simulink model "first_3phase_multilevel_doros"  (R2015a)
settings: Solver=ode45  StartTime=0.02  StopTime=0.04  RelTol=1e-3
libraries: simulink x85, powerlib_meascontrol x77, powerlib x52
settings Model: Creator=yahya  LastModifiedBy=Yahya

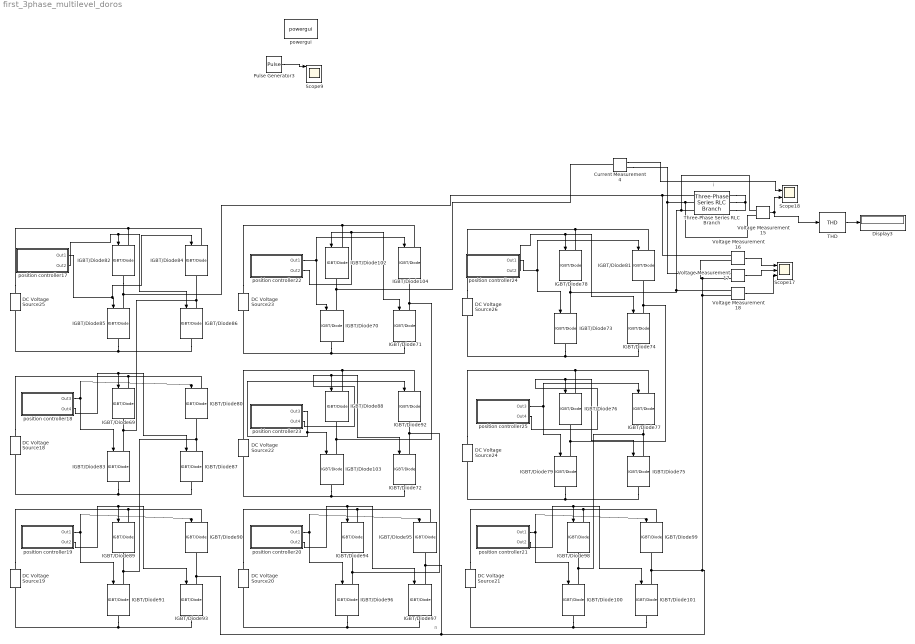
== system first_3phase_multilevel_doros ==
  note: n
  note: i
  Current Measurement4 : powerlib/Measurements/Current Measurement  PhasorSimulation=off  OutputType=Complex  PSBequivalent=0
  DC Voltage Source{18..26} (9 alike) : powerlib/Electrical Sources/DC Voltage Source  Amplitude=100  Measurements=None
  Display3 : Display
  IGBT/Diode{69..104} (36 alike) : powerlib/Power Electronics/IGBT//Diode  Ron=1e-3  Rs=1e5  Cs=inf  Measurements=off
  Pulse Generator3 : DiscretePulseGenerator  PulseType=Time based  Amplitude=0.8  Period=0.00001  PulseWidth=50
  Scope17 : Scope  NumInputPorts=3
      settings: TimeRange=0.02  YMin=-5~-5~-5  YMax=5~5~5  SaveName=ScopeData15
  Scope18 : Scope  NumInputPorts=2
      settings: TimeRange=1  YMin=-400~-400  YMax=400~400  SaveName=ScopeData16
  Scope9 : Scope  NumInputPorts=4
      settings: YMin=-5~-5~-5~-5  YMax=5~5~5~5  SaveName=ScopeData18
  THD : powerlib_meascontrol/Measurements/THD  Freq=50  Ts=0
  Three-Phase Series RLC Branch : powerlib/Elements/Three-Phase Series RLC Branch  LConnTagsString=A|B|C  RConnTagsString=A|B|C  BranchType=RL  Resistance=2.81  Inductance=0.01167  Capacitance=1e-6  Measurements=None
  Voltage Measurement{15..18} (4 alike) : powerlib/Measurements/Voltage Measurement  PhasorSimulation=off  OutputType=Complex  PSBequivalent=0
  position controller17 : Subsystem
  position controller18 : Subsystem
  position controller19 : Subsystem
  position controller20 : Subsystem
  position controller21 : Subsystem
  position controller22 : Subsystem
  position controller23 : Subsystem
  position controller24 : Subsystem
  position controller25 : Subsystem
  powergui : powerlib/powergui  Priority=1  SimulationMode=Continuous  SolverType=Tustin/Backward Euler (TBE)  SampleTime=50e-6  frequency=60  SPID=off  DisableSnubberDevices=off  DisableRonSwitches=off  DisableVfSwitches=off  SwTol=0  DisplayEquations=off  Interpol=off  methode=off  Ts=100  FunctionMessages=off  echomessages=off  HookPort=off  EnableUseOfTLC=off  x0status=blocks  frequencyindice=0  Pbase=100e6  ErrMax=1e-4  Iterations=50  UnitsV=kV  UnitsW=MW  buscounter=0  RestoreLinks=warning  ResistiveCurrentMeasurement=off  Frange=[0:2:500]  Ylog=off  Xlog=on  ShowGrid=off  save=off  variable=ZData  structure=0  ZoomFFT=off  StartTime=0.0  cycles=1  DisplayStyle=1  fundamental=60  FreqAxis=off  MaxFrequency=1000  frequencyindicesteady=1  RmsSteady=1  display=off
  wires:
  position controller17/2(Out2) -> IGBT/Diode86/1, IGBT/Diode82/1
  Pulse Generator3/1 -> Scope9/1
  Current Measurement4/1 -> Scope18/1
  position controller17/1(Out1) -> IGBT/Diode85/1, IGBT/Diode84/1
  position controller18/2(Out4) -> IGBT/Diode87/1, IGBT/Diode69/1
  position controller18/1(Out3) -> IGBT/Diode83/1, IGBT/Diode80/1
  position controller22/2(Out2) -> IGBT/Diode102/1, IGBT/Diode71/1
  position controller22/1(Out1) -> IGBT/Diode70/1, IGBT/Diode104/1
  position controller23/2(Out4) -> IGBT/Diode72/1, IGBT/Diode88/1
  position controller23/1(Out3) -> IGBT/Diode103/1, IGBT/Diode92/1
  position controller24/2(Out2) -> IGBT/Diode74/1, IGBT/Diode78/1
  position controller24/1(Out1) -> IGBT/Diode81/1, IGBT/Diode73/1
  position controller25/2(Out4) -> IGBT/Diode75/1, IGBT/Diode76/1
  position controller25/1(Out3) -> IGBT/Diode79/1, IGBT/Diode77/1
  Voltage Measurement15/1 -> Scope18/2, THD/1
  Voltage Measurement16/1 -> Scope17/1
  Voltage Measurement17/1 -> Scope17/2
  Voltage Measurement18/1 -> Scope17/3
  position controller19/2(Out2) -> IGBT/Diode93/1, IGBT/Diode89/1
  position controller19/1(Out1) -> IGBT/Diode91/1, IGBT/Diode90/1
  position controller20/2(Out2) -> IGBT/Diode97/1, IGBT/Diode94/1
  position controller20/1(Out1) -> IGBT/Diode96/1, IGBT/Diode95/1
  position controller21/2(Out2) -> IGBT/Diode101/1, IGBT/Diode98/1
  position controller21/1(Out1) -> IGBT/Diode100/1, IGBT/Diode99/1
  THD/1 -> Display3/1
  connections:
  DC Voltage Source25/RConn1 -- IGBT/Diode84/LConn1 -- IGBT/Diode82/LConn1
  DC Voltage Source25/LConn1 -- IGBT/Diode85/RConn1 -- IGBT/Diode86/RConn1
  IGBT/Diode84/RConn1 -- IGBT/Diode86/LConn1 -- IGBT/Diode69/RConn1 -- IGBT/Diode83/LConn1
  DC Voltage Source18/RConn1 -- IGBT/Diode80/LConn1 -- IGBT/Diode69/LConn1
  DC Voltage Source18/LConn1 -- IGBT/Diode87/RConn1 -- IGBT/Diode83/RConn1
  DC Voltage Source23/RConn1 -- IGBT/Diode104/LConn1 -- IGBT/Diode102/LConn1
  DC Voltage Source23/LConn1 -- IGBT/Diode71/RConn1 -- IGBT/Diode70/RConn1
  IGBT/Diode102/RConn1 -- Current Measurement4/LConn1 -- IGBT/Diode70/LConn1
  IGBT/Diode92/LConn1 -- DC Voltage Source22/RConn1 -- IGBT/Diode88/LConn1
  DC Voltage Source22/LConn1 -- IGBT/Diode72/RConn1 -- IGBT/Diode103/RConn1
  IGBT/Diode88/RConn1 -- IGBT/Diode103/LConn1 -- IGBT/Diode71/LConn1 -- IGBT/Diode104/RConn1
  DC Voltage Source26/RConn1 -- IGBT/Diode81/LConn1 -- IGBT/Diode78/LConn1
  DC Voltage Source26/LConn1 -- IGBT/Diode74/RConn1 -- IGBT/Diode73/RConn1
  DC Voltage Source24/RConn1 -- IGBT/Diode77/LConn1 -- IGBT/Diode76/LConn1
  DC Voltage Source24/LConn1 -- IGBT/Diode75/RConn1 -- IGBT/Diode79/RConn1
  IGBT/Diode74/LConn1 -- IGBT/Diode81/RConn1 -- IGBT/Diode76/RConn1 -- IGBT/Diode79/LConn1
  IGBT/Diode73/LConn1 -- Voltage Measurement15/LConn1 -- Three-Phase Series RLC Branch/LConn3 -- Voltage Measurement18/LConn1 -- IGBT/Diode78/RConn1
  IGBT/Diode82/RConn1 -- Three-Phase Series RLC Branch/LConn1 -- Voltage Measurement16/LConn1 -- IGBT/Diode85/LConn1
  Three-Phase Series RLC Branch/RConn2 -- Three-Phase Series RLC Branch/RConn3 -- Three-Phase Series RLC Branch/RConn1
  IGBT/Diode89/RConn1 -- IGBT/Diode91/LConn1 -- IGBT/Diode80/RConn1 -- IGBT/Diode87/LConn1
  IGBT/Diode94/RConn1 -- IGBT/Diode96/LConn1 -- IGBT/Diode92/RConn1 -- IGBT/Diode72/LConn1
  IGBT/Diode98/RConn1 -- IGBT/Diode100/LConn1 -- IGBT/Diode77/RConn1 -- IGBT/Diode75/LConn1
  DC Voltage Source19/RConn1 -- IGBT/Diode90/LConn1 -- IGBT/Diode89/LConn1
  DC Voltage Source19/LConn1 -- IGBT/Diode93/RConn1 -- IGBT/Diode91/RConn1
  DC Voltage Source20/RConn1 -- IGBT/Diode95/LConn1 -- IGBT/Diode94/LConn1
  DC Voltage Source20/LConn1 -- IGBT/Diode97/RConn1 -- IGBT/Diode96/RConn1
  DC Voltage Source21/RConn1 -- IGBT/Diode99/LConn1 -- IGBT/Diode98/LConn1
  DC Voltage Source21/LConn1 -- IGBT/Diode101/RConn1 -- IGBT/Diode100/RConn1
  IGBT/Diode93/LConn1 -- IGBT/Diode90/RConn1 -- Voltage Measurement16/LConn2 -- Voltage Measurement17/LConn2 -- Voltage Measurement18/LConn2 -- IGBT/Diode99/RConn1 -- IGBT/Diode101/LConn1 -- IGBT/Diode95/RConn1 -- IGBT/Diode97/LConn1
  Three-Phase Series RLC Branch/LConn2 -- Voltage Measurement17/LConn1 -- Current Measurement4/RConn1 -- Voltage Measurement15/LConn2

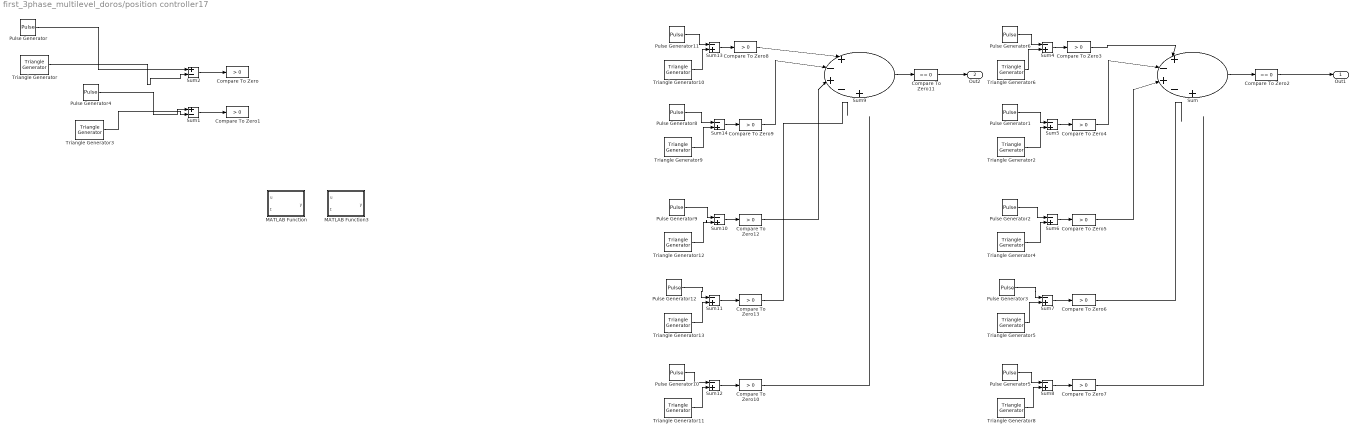
== system first_3phase_multilevel_doros/position controller17 ==
  Compare To Zero{,1,3..10,12..13} (12 alike) : simulink/Logic and Bit Operations/Compare To Zero  relop=>  OutDataTypeStr=boolean  ZeroCross=off
  Compare To Zero11 : simulink/Logic and Bit Operations/Compare To Zero  relop===  OutDataTypeStr=boolean  ZeroCross=off
  Compare To Zero2 : simulink/Logic and Bit Operations/Compare To Zero  relop===  OutDataTypeStr=boolean  ZeroCross=off
  MATLAB Function : MATLAB Function  TreatAsAtomicUnit=on
  MATLAB Function3 : MATLAB Function  TreatAsAtomicUnit=on
  Pulse Generator : DiscretePulseGenerator  PulseType=Time based  Amplitude=0.648099859976388  Period=0.02  PulseWidth=50.001
  Pulse Generator1 : DiscretePulseGenerator  PulseType=Time based  Amplitude=0.687674739965695  Period=0.02  PulseWidth=50.001
  Pulse Generator10 : DiscretePulseGenerator  PulseType=Time based  Amplitude=0.377812988041322  Period=0.02  PulseWidth=50.001  PhaseDelay=0.01
  Pulse Generator11 : DiscretePulseGenerator  PulseType=Time based  Amplitude=0.5150  Period=0.02  PulseWidth=50.001  PhaseDelay=0.01
  Pulse Generator12 : DiscretePulseGenerator  PulseType=Time based  Amplitude=0.360085258924687  Period=0.02  PulseWidth=50.001  PhaseDelay=0.01
  Pulse Generator2 : DiscretePulseGenerator  PulseType=Time based  Amplitude=0.796099800558993  Period=0.02  PulseWidth=50.001
  Pulse Generator3 : DiscretePulseGenerator  PulseType=Time based  Amplitude=0.360085258924687  Period=0.02  PulseWidth=50.001
  Pulse Generator4 : DiscretePulseGenerator  PulseType=Time based  Amplitude=0.648099859976388  Period=0.02  PulseWidth=50.001  PhaseDelay=0.01
  Pulse Generator5 : DiscretePulseGenerator  PulseType=Time based  Amplitude=0.377812988041322  Period=0.02  PulseWidth=50.001
  Pulse Generator6 : DiscretePulseGenerator  PulseType=Time based  Amplitude=0.5150  Period=0.02  PulseWidth=50.001
  Pulse Generator8 : DiscretePulseGenerator  PulseType=Time based  Amplitude=0.687674739965695  Period=0.02  PulseWidth=50.001  PhaseDelay=0.01
  Pulse Generator9 : DiscretePulseGenerator  PulseType=Time based  Amplitude=0.796099800558993  Period=0.02  PulseWidth=50.001  PhaseDelay=0.01
  Sum : Sum  Inputs=|+-+-+
  Sum1 : Sum  Inputs=+-  OutDataTypeStr=double
  Sum{4..8,10..14} (10 alike) : Sum  Inputs=-+  OutDataTypeStr=double
  Sum2 : Sum  Inputs=+-  OutDataTypeStr=double
  Sum9 : Sum  Inputs=|+-+-+
  Triangle Generator{,2,4..6,8} (6 alike) : powerlib_meascontrol/Pulse & Signal Generators/Triangle Generator  Freq=50  Phase=90  Ts=0
  Triangle Generator{3,9..13} (6 alike) : powerlib_meascontrol/Pulse & Signal Generators/Triangle Generator  Freq=50  Phase=90+180  Ts=0
  Out1 : Outport
  Out2 : Outport  Port=2
  wires:
  Pulse Generator/1 -> Sum2/1
  Triangle Generator/1 -> Sum2/2
  Pulse Generator4/1 -> Sum1/1
  Triangle Generator3/1 -> Sum1/2
  Sum2/1 -> Compare To Zero/1
  Sum1/1 -> Compare To Zero1/1
  Triangle Generator6/1 -> Sum4/2
  Sum4/1 -> Compare To Zero3/1
  Pulse Generator6/1 -> Sum4/1
  Triangle Generator2/1 -> Sum5/2
  Sum5/1 -> Compare To Zero4/1
  Pulse Generator1/1 -> Sum5/1
  Triangle Generator4/1 -> Sum6/2
  Sum6/1 -> Compare To Zero5/1
  Pulse Generator2/1 -> Sum6/1
  Triangle Generator5/1 -> Sum7/2
  Sum7/1 -> Compare To Zero6/1
  Pulse Generator3/1 -> Sum7/1
  Triangle Generator8/1 -> Sum8/2
  Sum8/1 -> Compare To Zero7/1
  Pulse Generator5/1 -> Sum8/1
  Compare To Zero3/1 -> Sum/1
  Compare To Zero5/1 -> Sum/3
  Compare To Zero6/1 -> ?
  Compare To Zero7/1 -> ?
  Triangle Generator10/1 -> Sum13/2
  Sum13/1 -> Compare To Zero8/1
  Pulse Generator11/1 -> Sum13/1
  Triangle Generator9/1 -> Sum14/2
  Sum14/1 -> Compare To Zero9/1
  Pulse Generator8/1 -> Sum14/1
  Triangle Generator12/1 -> Sum10/2
  Sum10/1 -> Compare To Zero12/1
  Pulse Generator9/1 -> Sum10/1
  Triangle Generator13/1 -> Sum11/2
  Sum11/1 -> Compare To Zero13/1
  Pulse Generator12/1 -> Sum11/1
  Triangle Generator11/1 -> Sum12/2
  Sum12/1 -> Compare To Zero10/1
  Pulse Generator10/1 -> Sum12/1
  Compare To Zero8/1 -> Sum9/1
  Compare To Zero9/1 -> Sum9/2
  Compare To Zero12/1 -> Sum9/3
  Sum9/1 -> Compare To Zero11/1
  Compare To Zero13/1 -> ?
  Compare To Zero10/1 -> ?
  Compare To Zero4/1 -> Sum/2
  Sum/1 -> Compare To Zero2/1
  Compare To Zero2/1 -> Out1/1
  Compare To Zero11/1 -> Out2/1

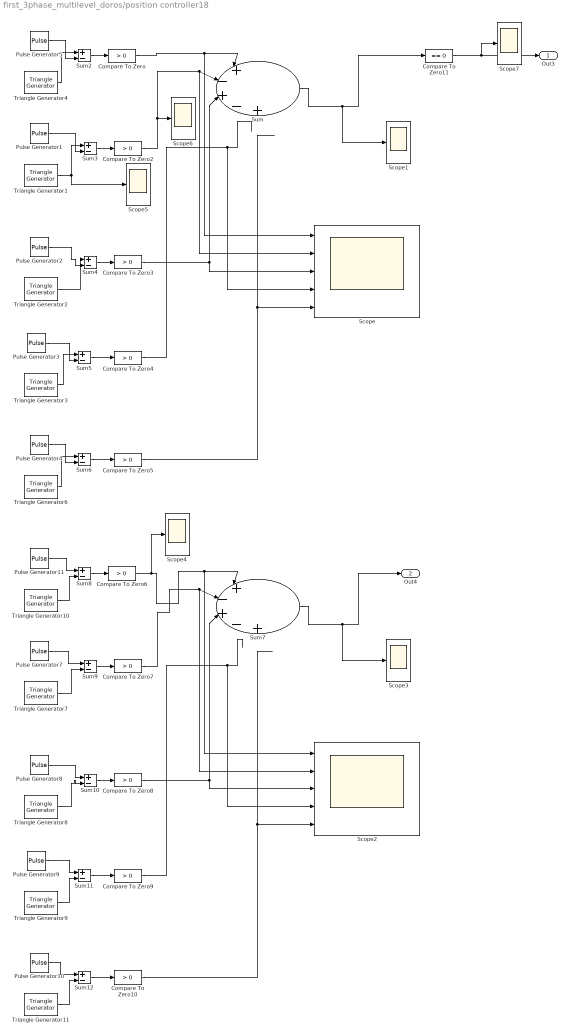
== system first_3phase_multilevel_doros/position controller18 ==
  Compare To Zero{,2..10} (10 alike) : simulink/Logic and Bit Operations/Compare To Zero  relop=>  OutDataTypeStr=boolean  ZeroCross=off
  Compare To Zero11 : simulink/Logic and Bit Operations/Compare To Zero  relop===  OutDataTypeStr=boolean  ZeroCross=off
  Pulse Generator1 : DiscretePulseGenerator  PulseType=Time based  Amplitude=0.372911525752630  Period=0.02  PulseWidth=50.001
  Pulse Generator10 : DiscretePulseGenerator  PulseType=Time based  Amplitude=0.377812988041322  Period=0.02  PulseWidth=50.001  PhaseDelay=0.01
  Pulse Generator11 : DiscretePulseGenerator  PulseType=Time based  Amplitude=0.3014  Period=0.02  PulseWidth=50.001  PhaseDelay=0.01
  Pulse Generator2 : DiscretePulseGenerator  PulseType=Time based  Amplitude=0.399283235379700  Period=0.02  PulseWidth=50.001
  Pulse Generator3 : DiscretePulseGenerator  PulseType=Time based  Amplitude=0.360085258924687  Period=0.02  PulseWidth=50.001
  Pulse Generator4 : DiscretePulseGenerator  PulseType=Time based  Amplitude=0.377812988041322  Period=0.02  PulseWidth=50.001
  Pulse Generator5 : DiscretePulseGenerator  PulseType=Time based  Amplitude=0.3014  Period=0.02  PulseWidth=50.001
  Pulse Generator7 : DiscretePulseGenerator  PulseType=Time based  Amplitude=0.372911525752630  Period=0.02  PulseWidth=50.001  PhaseDelay=0.01
  Pulse Generator8 : DiscretePulseGenerator  PulseType=Time based  Amplitude=0.399283235379700  Period=0.02  PulseWidth=50.001  PhaseDelay=0.01
  Pulse Generator9 : DiscretePulseGenerator  PulseType=Time based  Amplitude=0.360085258924687  Period=0.02  PulseWidth=50.001  PhaseDelay=0.01
  Scope : Scope  NumInputPorts=5
      settings: TimeRange=0.02  YMin=0~0~0~0~0  YMax=1~1~1~1~1  SaveName=ScopeData8
  Scope{1,3..7} (6 alike) : Scope
      Scope1 settings: SaveName=ScopeData17
      Scope3 settings: SaveName=ScopeData45
      Scope4 settings: SaveName=ScopeData46
      Scope5 settings: SaveName=ScopeData47
      Scope6 settings: SaveName=ScopeData48
      Scope7 settings: SaveName=ScopeData49
  Scope2 : Scope  NumInputPorts=5
      settings: YMin=-5~-5~-5~-5~-5  YMax=5~5~5~5~5  SaveName=ScopeData44
  Sum : Sum  Inputs=|+-+-+
  Sum{2..6,8..12} (10 alike) : Sum  Inputs=+-  OutDataTypeStr=double
  Sum7 : Sum  Inputs=|+-+-+
  Triangle Generator{1..4,6} (5 alike) : powerlib_meascontrol/Pulse & Signal Generators/Triangle Generator  Freq=50  Phase=90  Ts=0
  Triangle Generator{7..11} (5 alike) : powerlib_meascontrol/Pulse & Signal Generators/Triangle Generator  Freq=50  Phase=90+180  Ts=0
  Out3 : Outport
  Out4 : Outport  Port=2
  wires:
  Triangle Generator4/1 -> Sum2/1
  Sum2/1 -> Compare To Zero/1
  Pulse Generator5/1 -> Sum2/2
  Triangle Generator1/1 -> Sum3/1, Scope5/1
  Sum3/1 -> Compare To Zero2/1
  Pulse Generator1/1 -> Sum3/2
  Triangle Generator2/1 -> Sum4/1
  Sum4/1 -> Compare To Zero3/1
  Pulse Generator2/1 -> Sum4/2
  Triangle Generator3/1 -> Sum5/1
  Sum5/1 -> Compare To Zero4/1
  Pulse Generator3/1 -> Sum5/2
  Triangle Generator6/1 -> Sum6/1
  Sum6/1 -> Compare To Zero5/1
  Pulse Generator4/1 -> Sum6/2
  Compare To Zero/1 -> Scope/1, Sum/1
  Compare To Zero3/1 -> Sum/3, Scope/3
  Sum/1 -> Scope1/1, Compare To Zero11/1
  Compare To Zero4/1 -> Scope/4
  Compare To Zero5/1 -> Scope/5
  Triangle Generator10/1 -> Sum8/2
  Sum8/1 -> Compare To Zero6/1
  Pulse Generator11/1 -> Sum8/1
  Triangle Generator7/1 -> Sum9/2
  Sum9/1 -> Compare To Zero7/1
  Pulse Generator7/1 -> Sum9/1
  Triangle Generator8/1 -> Sum10/2
  Sum10/1 -> Compare To Zero8/1
  Pulse Generator8/1 -> Sum10/1
  Triangle Generator9/1 -> Sum11/2
  Sum11/1 -> Compare To Zero9/1
  Pulse Generator9/1 -> Sum11/1
  Triangle Generator11/1 -> Sum12/2
  Sum12/1 -> Compare To Zero10/1
  Pulse Generator10/1 -> Sum12/1
  Compare To Zero6/1 -> Scope4/1, Scope2/1, Sum7/1
  Compare To Zero7/1 -> Sum7/2, Scope2/2
  Compare To Zero8/1 -> Sum7/3, Scope2/3
  Sum7/1 -> Out4/1, Scope3/1
  Compare To Zero9/1 -> Scope2/4
  Compare To Zero10/1 -> Scope2/5
  Compare To Zero2/1 -> Sum/2, Scope/2, Scope6/1
  Compare To Zero11/1 -> Scope7/1, Out3/1

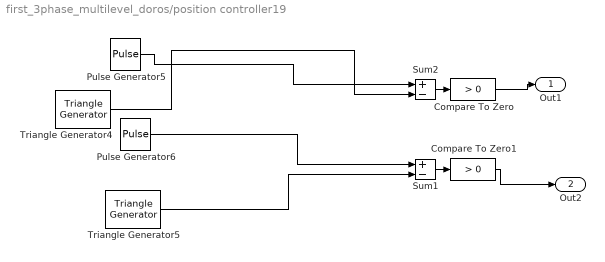
== system first_3phase_multilevel_doros/position controller19 ==
  Compare To Zero : simulink/Logic and Bit Operations/Compare To Zero  relop=>  OutDataTypeStr=boolean  ZeroCross=off
  Compare To Zero1 : simulink/Logic and Bit Operations/Compare To Zero  relop=>  OutDataTypeStr=boolean  ZeroCross=off
  Pulse Generator5 : DiscretePulseGenerator  PulseType=Time based  Amplitude=0.0158  Period=0.02  PulseWidth=50.001
  Pulse Generator6 : DiscretePulseGenerator  PulseType=Time based  Amplitude=0.0158  Period=0.02  PulseWidth=50.001  PhaseDelay=0.01
  Sum1 : Sum  Inputs=+-  OutDataTypeStr=double
  Sum2 : Sum  Inputs=+-  OutDataTypeStr=double
  Triangle Generator4 : powerlib_meascontrol/Pulse & Signal Generators/Triangle Generator  Freq=50  Phase=90  Ts=0
  Triangle Generator5 : powerlib_meascontrol/Pulse & Signal Generators/Triangle Generator  Freq=50  Phase=90+180  Ts=0
  Out1 : Outport
  Out2 : Outport  Port=2
  wires:
  Compare To Zero/1 -> Out1/1
  Compare To Zero1/1 -> Out2/1
  Pulse Generator5/1 -> Sum2/1
  Triangle Generator4/1 -> Sum2/2
  Pulse Generator6/1 -> Sum1/1
  Triangle Generator5/1 -> Sum1/2
  Sum2/1 -> Compare To Zero/1
  Sum1/1 -> Compare To Zero1/1

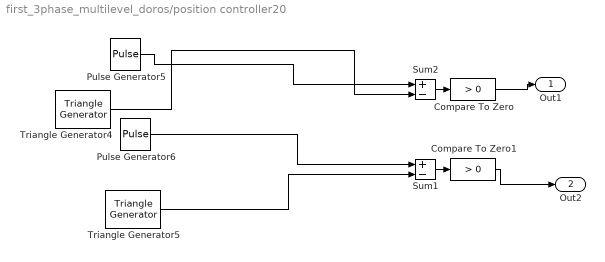
== system first_3phase_multilevel_doros/position controller20 ==
  Compare To Zero : simulink/Logic and Bit Operations/Compare To Zero  relop=>  OutDataTypeStr=boolean  ZeroCross=off
  Compare To Zero1 : simulink/Logic and Bit Operations/Compare To Zero  relop=>  OutDataTypeStr=boolean  ZeroCross=off
  Pulse Generator5 : DiscretePulseGenerator  PulseType=Time based  Amplitude=0.0158  Period=0.02  PulseWidth=50.001  PhaseDelay=0.006666666666667
  Pulse Generator6 : DiscretePulseGenerator  PulseType=Time based  Amplitude=0.0158  Period=0.02  PulseWidth=50.001  PhaseDelay=0.01+0.006666666666667
  Sum1 : Sum  Inputs=+-  OutDataTypeStr=double
  Sum2 : Sum  Inputs=+-  OutDataTypeStr=double
  Triangle Generator4 : powerlib_meascontrol/Pulse & Signal Generators/Triangle Generator  Freq=50  Phase=90+240  Ts=0
  Triangle Generator5 : powerlib_meascontrol/Pulse & Signal Generators/Triangle Generator  Freq=50  Phase=90+180+240  Ts=0
  Out1 : Outport
  Out2 : Outport  Port=2
  wires:
  Compare To Zero/1 -> Out1/1
  Compare To Zero1/1 -> Out2/1
  Pulse Generator5/1 -> Sum2/1
  Triangle Generator4/1 -> Sum2/2
  Pulse Generator6/1 -> Sum1/1
  Triangle Generator5/1 -> Sum1/2
  Sum2/1 -> Compare To Zero/1
  Sum1/1 -> Compare To Zero1/1

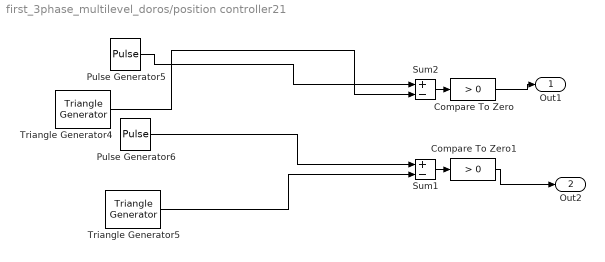
== system first_3phase_multilevel_doros/position controller21 ==
  Compare To Zero : simulink/Logic and Bit Operations/Compare To Zero  relop=>  OutDataTypeStr=boolean  ZeroCross=off
  Compare To Zero1 : simulink/Logic and Bit Operations/Compare To Zero  relop=>  OutDataTypeStr=boolean  ZeroCross=off
  Pulse Generator5 : DiscretePulseGenerator  PulseType=Time based  Amplitude=0.0158  Period=0.02  PulseWidth=50.001  PhaseDelay=0.013333333333333
  Pulse Generator6 : DiscretePulseGenerator  PulseType=Time based  Amplitude=0.0158  Period=0.02  PulseWidth=50.001  PhaseDelay=0.01+0.013333333333333
  Sum1 : Sum  Inputs=+-  OutDataTypeStr=double
  Sum2 : Sum  Inputs=+-  OutDataTypeStr=double
  Triangle Generator4 : powerlib_meascontrol/Pulse & Signal Generators/Triangle Generator  Freq=50  Phase=90+120  Ts=0
  Triangle Generator5 : powerlib_meascontrol/Pulse & Signal Generators/Triangle Generator  Freq=50  Phase=90+180+120  Ts=0
  Out1 : Outport
  Out2 : Outport  Port=2
  wires:
  Compare To Zero/1 -> Out1/1
  Compare To Zero1/1 -> Out2/1
  Pulse Generator5/1 -> Sum2/1
  Triangle Generator4/1 -> Sum2/2
  Pulse Generator6/1 -> Sum1/1
  Triangle Generator5/1 -> Sum1/2
  Sum2/1 -> Compare To Zero/1
  Sum1/1 -> Compare To Zero1/1

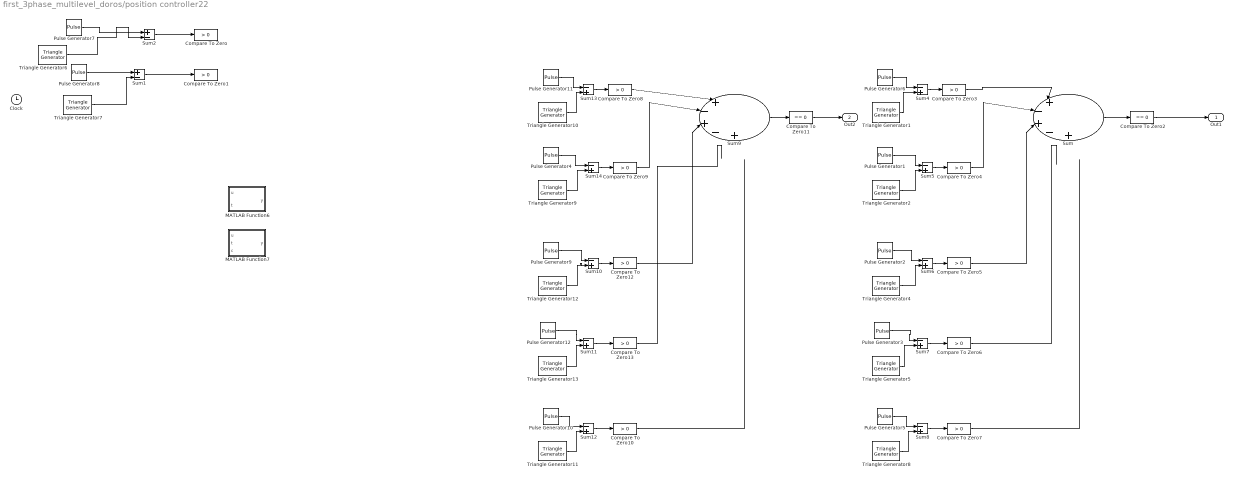
== system first_3phase_multilevel_doros/position controller22 ==
  Clock : Clock
  Compare To Zero{,1,3..10,12..13} (12 alike) : simulink/Logic and Bit Operations/Compare To Zero  relop=>  OutDataTypeStr=boolean  ZeroCross=off
  Compare To Zero11 : simulink/Logic and Bit Operations/Compare To Zero  relop===  OutDataTypeStr=boolean  ZeroCross=off
  Compare To Zero2 : simulink/Logic and Bit Operations/Compare To Zero  relop===  OutDataTypeStr=boolean  ZeroCross=off
  MATLAB Function6 : MATLAB Function  TreatAsAtomicUnit=on
  MATLAB Function7 : MATLAB Function  TreatAsAtomicUnit=on
  Pulse Generator1 : DiscretePulseGenerator  PulseType=Time based  Amplitude=0.687674739965695  Period=0.02  PulseWidth=50.001  PhaseDelay=0.006666666666667
  Pulse Generator10 : DiscretePulseGenerator  PulseType=Time based  Amplitude=0.377812988041322  Period=0.02  PulseWidth=50.001  PhaseDelay=0.01
  Pulse Generator11 : DiscretePulseGenerator  PulseType=Time based  Amplitude=0.5150  Period=0.02  PulseWidth=50.001  PhaseDelay=0.01+0.006666666666667
  Pulse Generator12 : DiscretePulseGenerator  PulseType=Time based  Amplitude=0.360085258924687  Period=0.02  PulseWidth=50.001  PhaseDelay=0.01
  Pulse Generator2 : DiscretePulseGenerator  PulseType=Time based  Amplitude=0.796099800558993  Period=0.02  PulseWidth=50.001  PhaseDelay=0.006666666666667
  Pulse Generator3 : DiscretePulseGenerator  PulseType=Time based  Amplitude=0.360085258924687  Period=0.02  PulseWidth=50.001
  Pulse Generator4 : DiscretePulseGenerator  PulseType=Time based  Amplitude=0.687674739965695  Period=0.02  PulseWidth=50.001  PhaseDelay=0.01+0.006666666666667
  Pulse Generator5 : DiscretePulseGenerator  PulseType=Time based  Amplitude=0.377812988041322  Period=0.02  PulseWidth=50.001
  Pulse Generator6 : DiscretePulseGenerator  PulseType=Time based  Amplitude=0.5150  Period=0.02  PulseWidth=50.001  PhaseDelay=0.006666666666667
  Pulse Generator7 : DiscretePulseGenerator  PulseType=Time based  Amplitude=0.648099859976388  Period=0.02  PulseWidth=50.001  PhaseDelay=0.006666666666667
  Pulse Generator8 : DiscretePulseGenerator  PulseType=Time based  Amplitude=0.648099859976388  Period=0.02  PulseWidth=50.001  PhaseDelay=0.01+0.006666666666667
  Pulse Generator9 : DiscretePulseGenerator  PulseType=Time based  Amplitude=0.796099800558993  Period=0.02  PulseWidth=50.001  PhaseDelay=0.01+0.006666666666667
  Sum : Sum  Inputs=|+-+-+
  Sum1 : Sum  Inputs=+-  OutDataTypeStr=double
  Sum{4..8,10..14} (10 alike) : Sum  Inputs=-+  OutDataTypeStr=double
  Sum2 : Sum  Inputs=+-  OutDataTypeStr=double
  Sum9 : Sum  Inputs=|+-+-+
  Triangle Generator{1..2,4,6} (4 alike) : powerlib_meascontrol/Pulse & Signal Generators/Triangle Generator  Freq=50  Phase=90+240  Ts=0
  Triangle Generator{7,9..10,12} (4 alike) : powerlib_meascontrol/Pulse & Signal Generators/Triangle Generator  Freq=50  Phase=90+180+240  Ts=0
  Triangle Generator11 : powerlib_meascontrol/Pulse & Signal Generators/Triangle Generator  Freq=50  Phase=90+180  Ts=0
  Triangle Generator13 : powerlib_meascontrol/Pulse & Signal Generators/Triangle Generator  Freq=50  Phase=90+180  Ts=0
  Triangle Generator5 : powerlib_meascontrol/Pulse & Signal Generators/Triangle Generator  Freq=50  Phase=90  Ts=0
  Triangle Generator8 : powerlib_meascontrol/Pulse & Signal Generators/Triangle Generator  Freq=50  Phase=90  Ts=0
  Out1 : Outport
  Out2 : Outport  Port=2
  wires:
  Triangle Generator6/1 -> Sum2/2
  Pulse Generator8/1 -> Sum1/1
  Pulse Generator7/1 -> Sum2/1
  Triangle Generator7/1 -> Sum1/2
  Sum2/1 -> Compare To Zero/1
  Sum1/1 -> Compare To Zero1/1
  Triangle Generator1/1 -> Sum4/2
  Sum4/1 -> Compare To Zero3/1
  Pulse Generator6/1 -> Sum4/1
  Triangle Generator2/1 -> Sum5/2
  Sum5/1 -> Compare To Zero4/1
  Pulse Generator1/1 -> Sum5/1
  Triangle Generator4/1 -> Sum6/2
  Sum6/1 -> Compare To Zero5/1
  Pulse Generator2/1 -> Sum6/1
  Triangle Generator5/1 -> Sum7/2
  Sum7/1 -> Compare To Zero6/1
  Pulse Generator3/1 -> Sum7/1
  Triangle Generator8/1 -> Sum8/2
  Sum8/1 -> Compare To Zero7/1
  Pulse Generator5/1 -> Sum8/1
  Compare To Zero3/1 -> Sum/1
  Compare To Zero5/1 -> Sum/3
  Compare To Zero6/1 -> ?
  Compare To Zero7/1 -> ?
  Triangle Generator10/1 -> Sum13/2
  Sum13/1 -> Compare To Zero8/1
  Pulse Generator11/1 -> Sum13/1
  Triangle Generator9/1 -> Sum14/2
  Sum14/1 -> Compare To Zero9/1
  Pulse Generator4/1 -> Sum14/1
  Triangle Generator12/1 -> Sum10/2
  Sum10/1 -> Compare To Zero12/1
  Pulse Generator9/1 -> Sum10/1
  Triangle Generator13/1 -> Sum11/2
  Sum11/1 -> Compare To Zero13/1
  Pulse Generator12/1 -> Sum11/1
  Triangle Generator11/1 -> Sum12/2
  Sum12/1 -> Compare To Zero10/1
  Pulse Generator10/1 -> Sum12/1
  Compare To Zero8/1 -> Sum9/1
  Compare To Zero9/1 -> Sum9/2
  Compare To Zero12/1 -> Sum9/3
  Sum9/1 -> Compare To Zero11/1
  Compare To Zero13/1 -> ?
  Compare To Zero10/1 -> ?
  Compare To Zero4/1 -> Sum/2
  Sum/1 -> Compare To Zero2/1
  Compare To Zero2/1 -> Out1/1
  Compare To Zero11/1 -> Out2/1

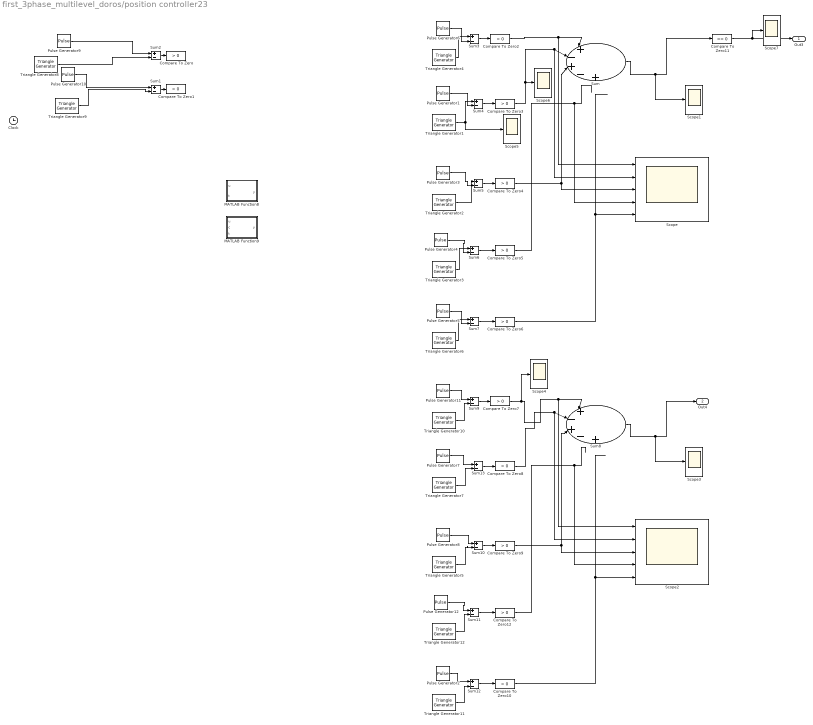
== system first_3phase_multilevel_doros/position controller23 ==
  Clock : Clock
  Compare To Zero{,1..10,12} (12 alike) : simulink/Logic and Bit Operations/Compare To Zero  relop=>  OutDataTypeStr=boolean  ZeroCross=off
  Compare To Zero11 : simulink/Logic and Bit Operations/Compare To Zero  relop===  OutDataTypeStr=boolean  ZeroCross=off
  MATLAB Function8 : MATLAB Function  TreatAsAtomicUnit=on
  MATLAB Function9 : MATLAB Function  TreatAsAtomicUnit=on
  Pulse Generator1 : DiscretePulseGenerator  PulseType=Time based  Amplitude=0.372911525752630  Period=0.02  PulseWidth=50.001  PhaseDelay=0.006666666666667
  Pulse Generator10 : DiscretePulseGenerator  PulseType=Time based  Amplitude=0.344892165427258  Period=0.02  PulseWidth=50.001  PhaseDelay=0.01+0.006666666666667
  Pulse Generator11 : DiscretePulseGenerator  PulseType=Time based  Amplitude=0.3014  Period=0.02  PulseWidth=50.001  PhaseDelay=0.01+0.006666666666667
  Pulse Generator12 : DiscretePulseGenerator  PulseType=Time based  Amplitude=0.360085258924687  Period=0.02  PulseWidth=50.001  PhaseDelay=0.01
  Pulse Generator2 : DiscretePulseGenerator  PulseType=Time based  Amplitude=0.377812988041322  Period=0.02  PulseWidth=50.001  PhaseDelay=0.01
  Pulse Generator3 : DiscretePulseGenerator  PulseType=Time based  Amplitude=0.399283235379700  Period=0.02  PulseWidth=50.001  PhaseDelay=0.006666666666667
  Pulse Generator4 : DiscretePulseGenerator  PulseType=Time based  Amplitude=0.360085258924687  Period=0.02  PulseWidth=50.001
  Pulse Generator5 : DiscretePulseGenerator  PulseType=Time based  Amplitude=0.377812988041322  Period=0.02  PulseWidth=50.001
  Pulse Generator6 : DiscretePulseGenerator  PulseType=Time based  Amplitude=0.3014  Period=0.02  PulseWidth=50.001  PhaseDelay=0.006666666666667
  Pulse Generator7 : DiscretePulseGenerator  PulseType=Time based  Amplitude=0.372911525752630  Period=0.02  PulseWidth=50.001  PhaseDelay=0.01+0.006666666666667
  Pulse Generator8 : DiscretePulseGenerator  PulseType=Time based  Amplitude=0.399283235379700  Period=0.02  PulseWidth=50.001  PhaseDelay=0.01+0.006666666666667
  Pulse Generator9 : DiscretePulseGenerator  PulseType=Time based  Amplitude=0.344892165427258  Period=0.02  PulseWidth=50.001  PhaseDelay=0.006666666666667
  Scope : Scope  NumInputPorts=5
      settings: TimeRange=0.02  YMin=0~0~0~0~0  YMax=1~1~1~1~1  SaveName=ScopeData50
  Scope{1,3..7} (6 alike) : Scope
      Scope1 settings: SaveName=ScopeData51
      Scope3 settings: SaveName=ScopeData53
      Scope4 settings: SaveName=ScopeData54
      Scope5 settings: SaveName=ScopeData55
      Scope6 settings: SaveName=ScopeData56
      Scope7 settings: SaveName=ScopeData57
  Scope2 : Scope  NumInputPorts=5
      settings: YMin=-5~-5~-5~-5~-5  YMax=5~5~5~5~5  SaveName=ScopeData52
  Sum : Sum  Inputs=|+-+-+
  Sum{1..7,9..13} (12 alike) : Sum  Inputs=+-  OutDataTypeStr=double
  Sum8 : Sum  Inputs=|+-+-+
  Triangle Generator{1..2,4,8} (4 alike) : powerlib_meascontrol/Pulse & Signal Generators/Triangle Generator  Freq=50  Phase=90+240  Ts=0
  Triangle Generator{5,7,9..10} (4 alike) : powerlib_meascontrol/Pulse & Signal Generators/Triangle Generator  Freq=50  Phase=90+180+240  Ts=0
  Triangle Generator11 : powerlib_meascontrol/Pulse & Signal Generators/Triangle Generator  Freq=50  Phase=90+180  Ts=0
  Triangle Generator12 : powerlib_meascontrol/Pulse & Signal Generators/Triangle Generator  Freq=50  Phase=90+180  Ts=0
  Triangle Generator3 : powerlib_meascontrol/Pulse & Signal Generators/Triangle Generator  Freq=50  Phase=90  Ts=0
  Triangle Generator6 : powerlib_meascontrol/Pulse & Signal Generators/Triangle Generator  Freq=50  Phase=90  Ts=0
  Out3 : Outport
  Out4 : Outport  Port=2
  wires:
  Triangle Generator8/1 -> Sum2/2
  Pulse Generator10/1 -> Sum1/1
  Triangle Generator9/1 -> Sum1/2
  Sum2/1 -> Compare To Zero/1
  Sum1/1 -> Compare To Zero1/1
  Pulse Generator9/1 -> Sum2/1
  Triangle Generator4/1 -> Sum3/1
  Sum3/1 -> Compare To Zero2/1
  Pulse Generator6/1 -> Sum3/2
  Triangle Generator1/1 -> Sum4/1, Scope5/1
  Sum4/1 -> Compare To Zero3/1
  Pulse Generator1/1 -> Sum4/2
  Triangle Generator2/1 -> Sum5/1
  Sum5/1 -> Compare To Zero4/1
  Pulse Generator3/1 -> Sum5/2
  Triangle Generator3/1 -> Sum6/1
  Sum6/1 -> Compare To Zero5/1
  Pulse Generator4/1 -> Sum6/2
  Triangle Generator6/1 -> Sum7/1
  Sum7/1 -> Compare To Zero6/1
  Pulse Generator5/1 -> Sum7/2
  Compare To Zero2/1 -> Scope/1, Sum/1
  Compare To Zero4/1 -> Sum/3, Scope/3
  Sum/1 -> Scope1/1, Compare To Zero11/1
  Compare To Zero5/1 -> Scope/4
  Compare To Zero6/1 -> Scope/5
  Triangle Generator10/1 -> Sum9/2
  Sum9/1 -> Compare To Zero7/1
  Pulse Generator11/1 -> Sum9/1
  Triangle Generator7/1 -> Sum13/2
  Sum13/1 -> Compare To Zero8/1
  Pulse Generator7/1 -> Sum13/1
  Triangle Generator5/1 -> Sum10/2
  Sum10/1 -> Compare To Zero9/1
  Pulse Generator8/1 -> Sum10/1
  Triangle Generator12/1 -> Sum11/2
  Sum11/1 -> Compare To Zero12/1
  Pulse Generator12/1 -> Sum11/1
  Triangle Generator11/1 -> Sum12/2
  Sum12/1 -> Compare To Zero10/1
  Pulse Generator2/1 -> Sum12/1
  Compare To Zero7/1 -> Scope4/1, Scope2/1, Sum8/1
  Compare To Zero8/1 -> Sum8/2, Scope2/2
  Compare To Zero9/1 -> Sum8/3, Scope2/3
  Sum8/1 -> Out4/1, Scope3/1
  Compare To Zero12/1 -> Scope2/4
  Compare To Zero10/1 -> Scope2/5
  Compare To Zero3/1 -> Sum/2, Scope/2, Scope6/1
  Compare To Zero11/1 -> Scope7/1, Out3/1

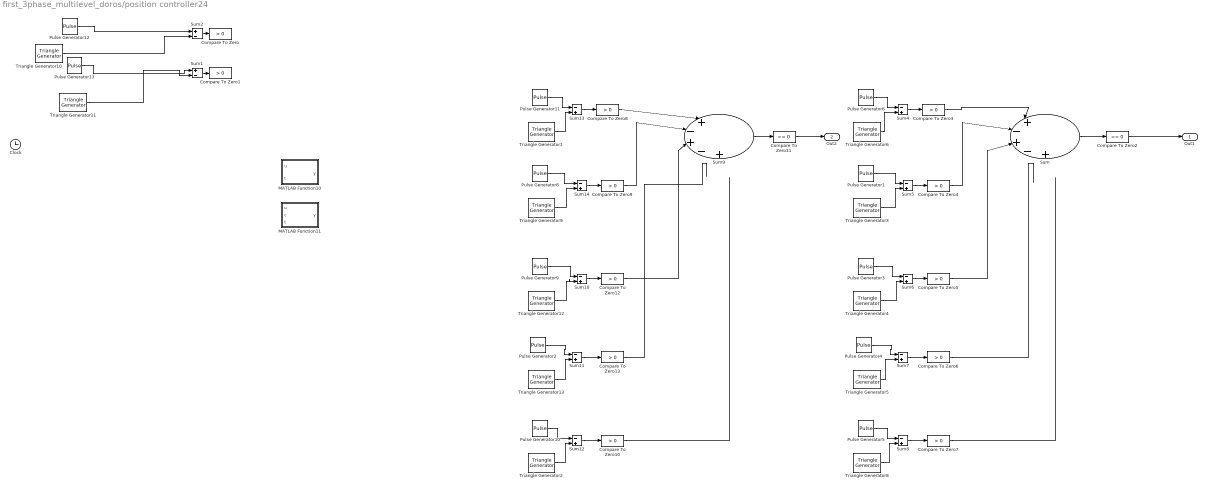
== system first_3phase_multilevel_doros/position controller24 ==
  Clock : Clock
  Compare To Zero{,1,3..10,12..13} (12 alike) : simulink/Logic and Bit Operations/Compare To Zero  relop=>  OutDataTypeStr=boolean  ZeroCross=off
  Compare To Zero11 : simulink/Logic and Bit Operations/Compare To Zero  relop===  OutDataTypeStr=boolean  ZeroCross=off
  Compare To Zero2 : simulink/Logic and Bit Operations/Compare To Zero  relop===  OutDataTypeStr=boolean  ZeroCross=off
  MATLAB Function10 : MATLAB Function  TreatAsAtomicUnit=on
  MATLAB Function11 : MATLAB Function  TreatAsAtomicUnit=on
  Pulse Generator1 : DiscretePulseGenerator  PulseType=Time based  Amplitude=0.687674739965695  Period=0.02  PulseWidth=50.001  PhaseDelay=0.013333333333333
  Pulse Generator10 : DiscretePulseGenerator  PulseType=Time based  Amplitude=0.377812988041322  Period=0.02  PulseWidth=50.001  PhaseDelay=0.01
  Pulse Generator11 : DiscretePulseGenerator  PulseType=Time based  Amplitude=0.5150  Period=0.02  PulseWidth=50.001  PhaseDelay=0.01+0.013333333333333
  Pulse Generator12 : DiscretePulseGenerator  PulseType=Time based  Amplitude=0.648099859976388  Period=0.02  PulseWidth=50.001  PhaseDelay=0.013333333333333
  Pulse Generator13 : DiscretePulseGenerator  PulseType=Time based  Amplitude=0.648099859976388  Period=0.02  PulseWidth=50.001  PhaseDelay=0.01+0.013333333333333
  Pulse Generator2 : DiscretePulseGenerator  PulseType=Time based  Amplitude=0.360085258924687  Period=0.02  PulseWidth=50.001  PhaseDelay=0.01
  Pulse Generator3 : DiscretePulseGenerator  PulseType=Time based  Amplitude=0.796099800558993  Period=0.02  PulseWidth=50.001  PhaseDelay=0.013333333333333
  Pulse Generator4 : DiscretePulseGenerator  PulseType=Time based  Amplitude=0.360085258924687  Period=0.02  PulseWidth=50.001
  Pulse Generator5 : DiscretePulseGenerator  PulseType=Time based  Amplitude=0.377812988041322  Period=0.02  PulseWidth=50.001
  Pulse Generator6 : DiscretePulseGenerator  PulseType=Time based  Amplitude=0.5150  Period=0.02  PulseWidth=50.001  PhaseDelay=0.013333333333333
  Pulse Generator8 : DiscretePulseGenerator  PulseType=Time based  Amplitude=0.687674739965695  Period=0.02  PulseWidth=50.001  PhaseDelay=0.01+0.013333333333333
  Pulse Generator9 : DiscretePulseGenerator  PulseType=Time based  Amplitude=0.796099800558993  Period=0.02  PulseWidth=50.001  PhaseDelay=0.01+0.013333333333333
  Sum : Sum  Inputs=|+-+-+
  Sum1 : Sum  Inputs=+-  OutDataTypeStr=double
  Sum{4..8,10..14} (10 alike) : Sum  Inputs=-+  OutDataTypeStr=double
  Sum2 : Sum  Inputs=+-  OutDataTypeStr=double
  Sum9 : Sum  Inputs=|+-+-+
  Triangle Generator{1,9,11..12} (4 alike) : powerlib_meascontrol/Pulse & Signal Generators/Triangle Generator  Freq=50  Phase=90+180+120  Ts=0
  Triangle Generator{3..4,6,10} (4 alike) : powerlib_meascontrol/Pulse & Signal Generators/Triangle Generator  Freq=50  Phase=90+120  Ts=0
  Triangle Generator13 : powerlib_meascontrol/Pulse & Signal Generators/Triangle Generator  Freq=50  Phase=90+180  Ts=0
  Triangle Generator2 : powerlib_meascontrol/Pulse & Signal Generators/Triangle Generator  Freq=50  Phase=90+180  Ts=0
  Triangle Generator5 : powerlib_meascontrol/Pulse & Signal Generators/Triangle Generator  Freq=50  Phase=90  Ts=0
  Triangle Generator8 : powerlib_meascontrol/Pulse & Signal Generators/Triangle Generator  Freq=50  Phase=90  Ts=0
  Out1 : Outport
  Out2 : Outport  Port=2
  wires:
  Triangle Generator10/1 -> Sum2/2
  Pulse Generator13/1 -> Sum1/1
  Triangle Generator11/1 -> Sum1/2
  Pulse Generator12/1 -> Sum2/1
  Sum2/1 -> Compare To Zero/1
  Sum1/1 -> Compare To Zero1/1
  Triangle Generator6/1 -> Sum4/2
  Sum4/1 -> Compare To Zero3/1
  Pulse Generator6/1 -> Sum4/1
  Triangle Generator3/1 -> Sum5/2
  Sum5/1 -> Compare To Zero4/1
  Pulse Generator1/1 -> Sum5/1
  Triangle Generator4/1 -> Sum6/2
  Sum6/1 -> Compare To Zero5/1
  Pulse Generator3/1 -> Sum6/1
  Triangle Generator5/1 -> Sum7/2
  Sum7/1 -> Compare To Zero6/1
  Pulse Generator4/1 -> Sum7/1
  Triangle Generator8/1 -> Sum8/2
  Sum8/1 -> Compare To Zero7/1
  Pulse Generator5/1 -> Sum8/1
  Compare To Zero3/1 -> Sum/1
  Compare To Zero5/1 -> Sum/3
  Compare To Zero6/1 -> ?
  Compare To Zero7/1 -> ?
  Triangle Generator1/1 -> Sum13/2
  Sum13/1 -> Compare To Zero8/1
  Pulse Generator11/1 -> Sum13/1
  Triangle Generator9/1 -> Sum14/2
  Sum14/1 -> Compare To Zero9/1
  Pulse Generator8/1 -> Sum14/1
  Triangle Generator12/1 -> Sum10/2
  Sum10/1 -> Compare To Zero12/1
  Pulse Generator9/1 -> Sum10/1
  Triangle Generator13/1 -> Sum11/2
  Sum11/1 -> Compare To Zero13/1
  Pulse Generator2/1 -> Sum11/1
  Triangle Generator2/1 -> Sum12/2
  Sum12/1 -> Compare To Zero10/1
  Pulse Generator10/1 -> Sum12/1
  Compare To Zero8/1 -> Sum9/1
  Compare To Zero9/1 -> Sum9/2
  Compare To Zero12/1 -> Sum9/3
  Sum9/1 -> Compare To Zero11/1
  Compare To Zero13/1 -> ?
  Compare To Zero10/1 -> ?
  Compare To Zero4/1 -> Sum/2
  Sum/1 -> Compare To Zero2/1
  Compare To Zero2/1 -> Out1/1
  Compare To Zero11/1 -> Out2/1

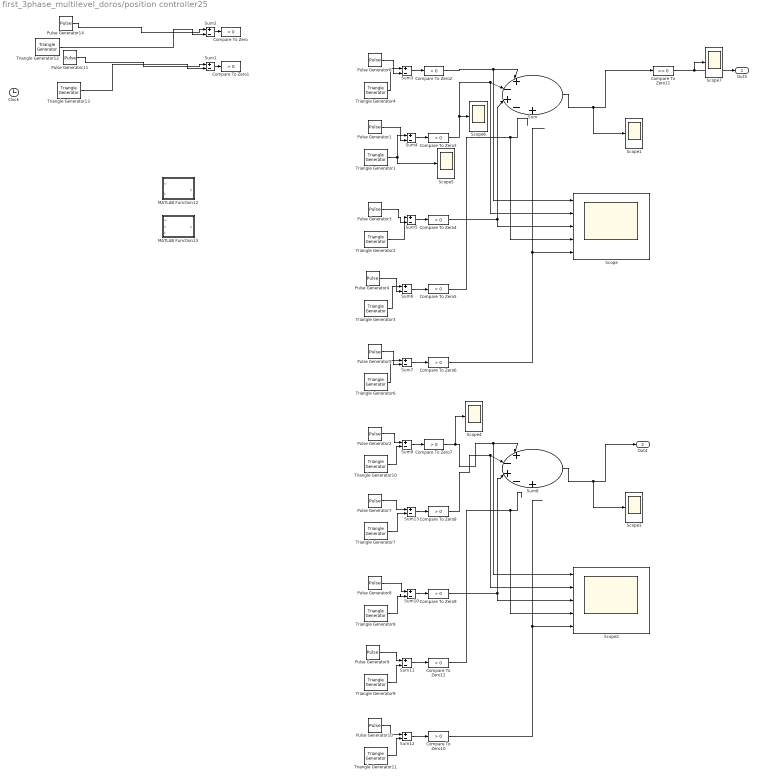
== system first_3phase_multilevel_doros/position controller25 ==
  Clock : Clock
  Compare To Zero{,1..10,12} (12 alike) : simulink/Logic and Bit Operations/Compare To Zero  relop=>  OutDataTypeStr=boolean  ZeroCross=off
  Compare To Zero11 : simulink/Logic and Bit Operations/Compare To Zero  relop===  OutDataTypeStr=boolean  ZeroCross=off
  MATLAB Function12 : MATLAB Function  TreatAsAtomicUnit=on
  MATLAB Function13 : MATLAB Function  TreatAsAtomicUnit=on
  Pulse Generator1 : DiscretePulseGenerator  PulseType=Time based  Amplitude=0.372911525752630  Period=0.02  PulseWidth=50.001  PhaseDelay=0.013333333333333
  Pulse Generator10 : DiscretePulseGenerator  PulseType=Time based  Amplitude=0.377812988041322  Period=0.02  PulseWidth=50.001  PhaseDelay=0.01
  Pulse Generator11 : DiscretePulseGenerator  PulseType=Time based  Amplitude=0.344892165427258  Period=0.02  PulseWidth=50.001  PhaseDelay=0.01+0.013333333333333
  Pulse Generator14 : DiscretePulseGenerator  PulseType=Time based  Amplitude=0.344892165427258  Period=0.02  PulseWidth=50.001  PhaseDelay=0.013333333333333
  Pulse Generator2 : DiscretePulseGenerator  PulseType=Time based  Amplitude=0.3014  Period=0.02  PulseWidth=50.001  PhaseDelay=0.01+0.013333333333333
  Pulse Generator3 : DiscretePulseGenerator  PulseType=Time based  Amplitude=0.399283235379700  Period=0.02  PulseWidth=50.001  PhaseDelay=0.013333333333333
  Pulse Generator4 : DiscretePulseGenerator  PulseType=Time based  Amplitude=0.360085258924687  Period=0.02  PulseWidth=50.001
  Pulse Generator5 : DiscretePulseGenerator  PulseType=Time based  Amplitude=0.377812988041322  Period=0.02  PulseWidth=50.001
  Pulse Generator6 : DiscretePulseGenerator  PulseType=Time based  Amplitude=0.3014  Period=0.02  PulseWidth=50.001  PhaseDelay=0.013333333333333
  Pulse Generator7 : DiscretePulseGenerator  PulseType=Time based  Amplitude=0.372911525752630  Period=0.02  PulseWidth=50.001  PhaseDelay=0.01+0.013333333333333
  Pulse Generator8 : DiscretePulseGenerator  PulseType=Time based  Amplitude=0.399283235379700  Period=0.02  PulseWidth=50.001  PhaseDelay=0.01+0.013333333333333
  Pulse Generator9 : DiscretePulseGenerator  PulseType=Time based  Amplitude=0.360085258924687  Period=0.02  PulseWidth=50.001  PhaseDelay=0.01
  Scope : Scope  NumInputPorts=5
      settings: TimeRange=0.02  YMin=0~0~0~0~0  YMax=1~1~1~1~1  SaveName=ScopeData58
  Scope{1,3..7} (6 alike) : Scope
      Scope1 settings: SaveName=ScopeData59
      Scope3 settings: SaveName=ScopeData61
      Scope4 settings: SaveName=ScopeData62
      Scope5 settings: SaveName=ScopeData63
      Scope6 settings: SaveName=ScopeData64
      Scope7 settings: SaveName=ScopeData65
  Scope2 : Scope  NumInputPorts=5
      settings: YMin=-5~-5~-5~-5~-5  YMax=5~5~5~5~5  SaveName=ScopeData60
  Sum : Sum  Inputs=|+-+-+
  Sum{1..7,9..13} (12 alike) : Sum  Inputs=+-  OutDataTypeStr=double
  Sum8 : Sum  Inputs=|+-+-+
  Triangle Generator{1..2,4,12} (4 alike) : powerlib_meascontrol/Pulse & Signal Generators/Triangle Generator  Freq=50  Phase=90+120  Ts=0
  Triangle Generator{7..8,10,13} (4 alike) : powerlib_meascontrol/Pulse & Signal Generators/Triangle Generator  Freq=50  Phase=90+180+120  Ts=0
  Triangle Generator11 : powerlib_meascontrol/Pulse & Signal Generators/Triangle Generator  Freq=50  Phase=90+180  Ts=0
  Triangle Generator3 : powerlib_meascontrol/Pulse & Signal Generators/Triangle Generator  Freq=50  Phase=90  Ts=0
  Triangle Generator6 : powerlib_meascontrol/Pulse & Signal Generators/Triangle Generator  Freq=50  Phase=90  Ts=0
  Triangle Generator9 : powerlib_meascontrol/Pulse & Signal Generators/Triangle Generator  Freq=50  Phase=90+180  Ts=0
  Out3 : Outport
  Out4 : Outport  Port=2
  wires:
  Pulse Generator14/1 -> Sum2/1
  Triangle Generator12/1 -> Sum2/2
  Pulse Generator11/1 -> Sum1/1
  Triangle Generator13/1 -> Sum1/2
  Sum2/1 -> Compare To Zero/1
  Sum1/1 -> Compare To Zero1/1
  Triangle Generator4/1 -> Sum3/1
  Sum3/1 -> Compare To Zero2/1
  Pulse Generator6/1 -> Sum3/2
  Triangle Generator1/1 -> Sum4/1, Scope5/1
  Sum4/1 -> Compare To Zero3/1
  Pulse Generator1/1 -> Sum4/2
  Triangle Generator2/1 -> Sum5/1
  Sum5/1 -> Compare To Zero4/1
  Pulse Generator3/1 -> Sum5/2
  Triangle Generator3/1 -> Sum6/1
  Sum6/1 -> Compare To Zero5/1
  Pulse Generator4/1 -> Sum6/2
  Triangle Generator6/1 -> Sum7/1
  Sum7/1 -> Compare To Zero6/1
  Pulse Generator5/1 -> Sum7/2
  Compare To Zero2/1 -> Scope/1, Sum/1
  Compare To Zero4/1 -> Sum/3, Scope/3
  Sum/1 -> Scope1/1, Compare To Zero11/1
  Compare To Zero5/1 -> Scope/4
  Compare To Zero6/1 -> Scope/5
  Triangle Generator10/1 -> Sum9/2
  Sum9/1 -> Compare To Zero7/1
  Pulse Generator2/1 -> Sum9/1
  Triangle Generator7/1 -> Sum13/2
  Sum13/1 -> Compare To Zero8/1
  Pulse Generator7/1 -> Sum13/1
  Triangle Generator8/1 -> Sum10/2
  Sum10/1 -> Compare To Zero9/1
  Pulse Generator8/1 -> Sum10/1
  Triangle Generator9/1 -> Sum11/2
  Sum11/1 -> Compare To Zero12/1
  Pulse Generator9/1 -> Sum11/1
  Triangle Generator11/1 -> Sum12/2
  Sum12/1 -> Compare To Zero10/1
  Pulse Generator10/1 -> Sum12/1
  Compare To Zero7/1 -> Scope4/1, Scope2/1, Sum8/1
  Compare To Zero8/1 -> Sum8/2, Scope2/2
  Compare To Zero9/1 -> Sum8/3, Scope2/3
  Sum8/1 -> Out4/1, Scope3/1
  Compare To Zero12/1 -> Scope2/4
  Compare To Zero10/1 -> Scope2/5
  Compare To Zero3/1 -> Sum/2, Scope/2, Scope6/1
  Compare To Zero11/1 -> Scope7/1, Out3/1

== matlab function first_3phase_multilevel_doros/position controller17/MATLAB Function ==
  data: u input; y output; t input
function y = fcn(u,t)
%#codegen
if t>u
    y = 1;
else
    y = 0;
end
end

== matlab function first_3phase_multilevel_doros/position controller17/MATLAB Function3 ==
  data: u input; y output; t input
function y = fcn(u,t)
%#codegen
if t>u
    y = 1;
else
    y = 0;
end
end

== matlab function first_3phase_multilevel_doros/position controller22/MATLAB Function6 ==
  data: u input; y output; t input
function y = fcn(u,t)
%#codegen
if t>u
    y = 1;
else
    y = 0;
end
end

== matlab function first_3phase_multilevel_doros/position controller22/MATLAB Function7 ==
  data: u input; y output; t input; c input
function y = fcn(u,t,c)
%#codegen
if t>u
    y = 1;
else
    y = 0;
end
if c<0.02
    y =0;
end

== matlab function first_3phase_multilevel_doros/position controller23/MATLAB Function8 ==
  data: u input; y output; t input
function y = fcn(u,t)
%#codegen
if t>u
    y = 1;
else
    y = 0;
end
end

== matlab function first_3phase_multilevel_doros/position controller23/MATLAB Function9 ==
  data: u input; c input; y output; t input
function y = fcn(u,c,t)
%#codegen
if t>u
    y = 1;
else
    y = 0;
end
if c <0.02
    y = 0;
end

== matlab function first_3phase_multilevel_doros/position controller24/MATLAB Function10 ==
  data: u input; y output; t input
function y = fcn(u,t)
%#codegen
if t>u
    y = 1;
else
    y = 0;
end
end

== matlab function first_3phase_multilevel_doros/position controller24/MATLAB Function11 ==
  data: u input; c input; y output; t input
function y = fcn(u,c,t)
%#codegen
if t>u
    y = 1;
else
    y = 0;
end
if c<0.02
    y = 0;
end

== matlab function first_3phase_multilevel_doros/position controller25/MATLAB Function12 ==
  data: u input; y output; t input
function y = fcn(u,t)
%#codegen
if t>u
    y = 1;
else
    y = 0;
end
end

== matlab function first_3phase_multilevel_doros/position controller25/MATLAB Function13 ==
  data: u input; c input; y output; t input
function y = fcn(u,c,t)
%#codegen
if t>u
    y = 1;
else
    y = 0;
end
if c<0.02
    y = 0;
end
